simulink model "dvbs1_batch"  (R2024b)
settings: Solver=VariableStepDiscrete  StartTime=0.0  StopTime=inf  RelTol=1e-3  EnableMultiTasking=on
values from neighbouring files (symbols this model uses):
  EbNo = 3.3    [errPattern.m]    (also in symuluj_przeplot.m = 0:0.1:2.9)
  M = 4    [errPattern.m]    (also in wsp_szczytu.m)
undefined symbols (not defined in the file or in its folder): EbNodB, rsgenpoly
libraries: simulink x4, commsink2 x3, commdigbbndpm3 x3, commblkcod2 x2, commcnvcod2 x2, commcnvintrlv2 x2, commchan3 x1, commrandsrc2 x1
settings Model: Creator=Administrator  LastModifiedBy=mateu
settings SolverCC: AlgebraicLoopSolver=TrustRegion
settings DataIOCC: LimitDataPoints=on  SaveFormat=Array  SignalLoggingSaveFormat=ModelDataLogs  ReturnWorkspaceOutputs=off
settings OptimizationCC: ExpressionDepthLimit=2147483647  InitFltsAndDblsToZero=on  LifeSpan=inf
settings DebuggingCC: UnderspecifiedInitializationDetection=Classic  MergeDetectMultiDrivingBlocksExec=none  SolverPrmCheckMsg=warning  FcnCallInpInsideContextMsg=warning  UnconnectedInputMsg=warning  UnconnectedOutputMsg=warning  UnconnectedLineMsg=warning  StateNameClashWarn=warning  SFUnexpectedBacktrackingDiag=warning  SFNoUnconditionalDefaultTransitionDiag=warning  ArithmeticOperatorsInVariantConditions=warning
settings HardwareCC: ProdBitPerPointer=32  ProdBitPerSizeT=32  ProdBitPerPtrDiffT=32  ProdLargestAtomicFloat=None  ProdIntDivRoundTo=Undefined  ProdEndianess=Unspecified  ProdWordSize=32  ProdHWDeviceType=32-bit Generic
settings ModelReferenceCC: EnableRefExpFcnMdlSchedulingChecks=on  PropagateSignalLabelsOutOfModel=off
settings SFSimCC: SimUseLocalCustomCode=off  CustomCodeUndefinedFunction=UseInterfaceOnly
settings RTWCC: RTWUseLocalCustomCode=off  GPUComputeCapability=3.5
settings CodeAppCC: StateflowObjectComments=on
settings GRTTargetCC: TargetLangStandard=C89/C90 (ANSI)  CombineOutputUpdateFcns=off  GRTInterface=on
settings ConfigComp: CovMetricSettings=dw  CovSaveCumulativeToWorkspaceVar=on  CovSaveSingleToWorkspaceVar=on  CovExternalEMLEnable=off  CovSFcnEnable=off

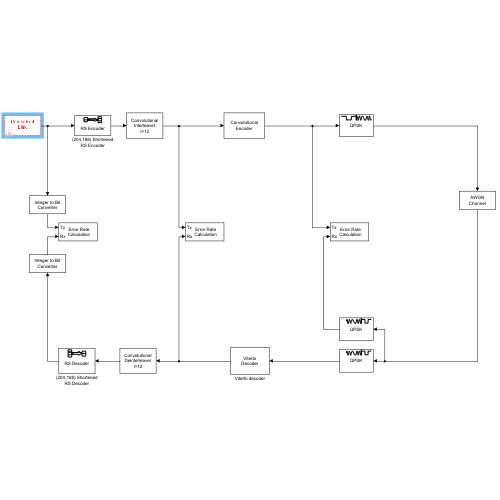
[thumbnail: Simulink's stored preview of the top-level diagram]
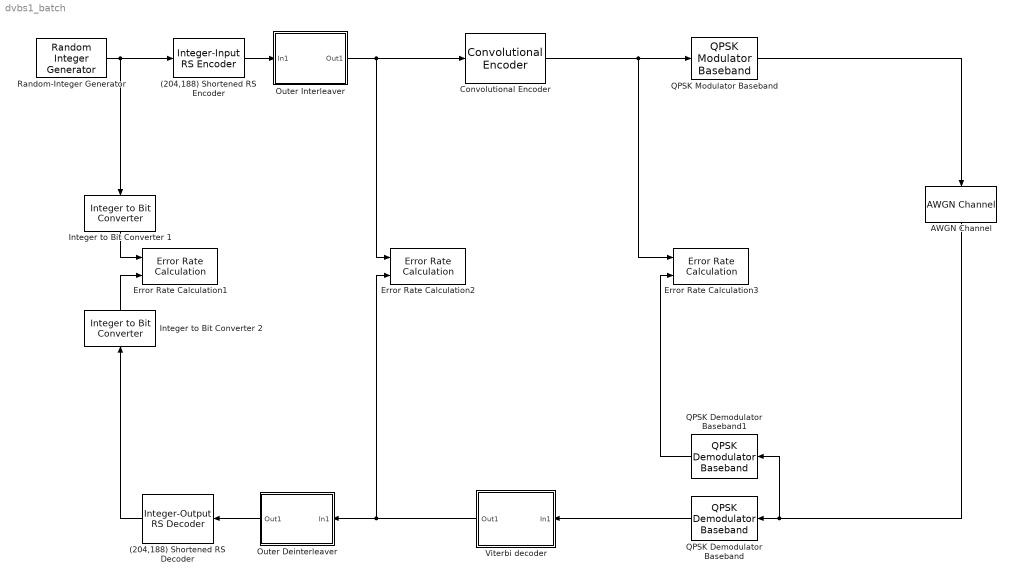
== system dvbs1_batch ==
  (204,188) Shortened RS Decoder : commblkcod2/Integer-Output RS Decoder  n=204  k=188  specShortening=off  shortenedK=3  specGenPoly=off  genPoly=rsgenpoly(7,3)  specPrimPoly=off  prPoly=[1 0 1 1]  specPuncture=off  punctVec=[ones(2,1); zeros(2,1)]  specErasurePort=off  showNumErr=off
  (204,188) Shortened RS Encoder : commblkcod2/Integer-Input RS Encoder  n=204  k=188  specShortening=off  shortenedK=3  specGenPoly=off  genPoly=rsgenpoly(7,3)  specPrimPoly=off  prPoly=[1 0 1 1]  specPuncture=off  punctVec=[ones(2,1); zeros(2,1)]
  AWGN Channel : commchan3/AWGN Channel  LegacyMode=on  NoiseMethod="Signal to noise ratio  (SNR)"  noiseMode="Signal to noise ratio  (SNR)"  EbNo=EbNo  EsNo=EbNodB+10*log10(log2(M))  SNR=EbNo + 1.20574  BitsPerSymbol=2  SignalPower=1  SamplesPerSymbol=1  SymbolPeriod=1.334  VarianceSource=Parameter  Variance=10^(-0.1*15)/(2048*2)  RandomStream=Global stream  Seed=54321  SimulateUsing=Code generation
  Convolutional Encoder : commcnvcod2/Convolutional Encoder  trellis=poly2trellis(7, [171 133])  opMode=Continuous  DelayedResetAction=off  hasIniStPort=off  hasFinStPort=off  usePuncVector=on  punctureVector=[1; 1; 0; 1]  reset=Unused parameter value
  Error Rate Calculation1 : commsink2/Error Rate Calculation  N=1504  st_delay=0  cp_mode=Entire frame  subframe=[]  PMode=Workspace  WsName=BerRs  RsMode2=off  stop=on  numErr=100  maxBits=1e7
  Error Rate Calculation2 : commsink2/Error Rate Calculation  N=1632  st_delay=0  cp_mode=Entire frame  subframe=[]  PMode=Workspace  WsName=BerFec  RsMode2=off  stop=off  numErr=100  maxBits=1e8
  Error Rate Calculation3 : commsink2/Error Rate Calculation  N=0  st_delay=0  cp_mode=Entire frame  subframe=[]  PMode=Workspace  WsName=BerRaw  RsMode2=off  stop=off  numErr=100  maxBits=1e8
  Integer to Bit Converter 1 : simulink/Logic and Bit Operations/Integer to Bit Converter  nbits=8  signedInputValues=Unsigned  bitOrder=MSB first  outDtype=boolean
  Integer to Bit Converter 2 : simulink/Logic and Bit Operations/Integer to Bit Converter  nbits=8  signedInputValues=Unsigned  bitOrder=MSB first  outDtype=boolean
  Outer Deinterleaver : Subsystem  mask(Convolutional Deinterleaver){}
      mask Display: disp('Convolutional\nDeinterleaver\nI=12')
  Outer Interleaver : Subsystem  mask(Convolutional Interleaver){}
      mask Display: disp('Convolutional\nInterleaver\nI=12')
  QPSK Demodulator Baseband : commdigbbndpm3/QPSK Demodulator Baseband  OutType=Bit  DecType=Approximate log-likelihood ratio  VarSource=Dialog  Variance=(1.0/(2*0.66))*10^(-EbNo/10)  Dec=Gray  Ph=pi/4  outDtype1=boolean  outDtype2=Inherit via internal rule  derotateFactorWordLen=16  derotateFactorDataTypeStr=Inherit: Same word length as input  derotateFactorLastDataTypeStr=Inherit: Same word length as input
  QPSK Demodulator Baseband1 : commdigbbndpm3/QPSK Demodulator Baseband  OutType=Bit  DecType=Hard decision  VarSource=Dialog  Variance=(1.0/(2*0.66))*10^(-EbNo/10)  Dec=Gray  Ph=pi/4  outDtype1=boolean  outDtype2=Inherit via internal rule  derotateFactorWordLen=16  derotateFactorDataTypeStr=Inherit: Same word length as input  derotateFactorLastDataTypeStr=Inherit: Same word length as input
  QPSK Modulator Baseband : commdigbbndpm3/QPSK Modulator Baseband  InType=Bit  Enc=Gray  Ph=pi/4  outDtype=double  outWordLen=16  outUDDataType=sfix(16)  outFracLenMode=Best precision  outFracLen=15  outDataTypeStr=double  outLastDataTypeStr=double
  Random-Integer Generator : commrandsrc2/Random Integer Generator  mul=256  seed=1234573  Ts=8*(204/188)  frameBased=on  sampPerFrame=188  orient=off  outDataType=uint8
  Viterbi decoder : Subsystem
      mask Display: disp('Viterbi\nDecoder')
  wires:
  (204,188) Shortened RS Encoder/1 -> Outer Interleaver/1(In1)
  Outer Interleaver/1(Out1) -> Convolutional Encoder/1, Error Rate Calculation2/1
  QPSK Modulator Baseband/1 -> AWGN Channel/1
  QPSK Demodulator Baseband/1 -> Viterbi decoder/1(In1)
  Outer Deinterleaver/1(Out1) -> (204,188) Shortened RS Decoder/1
  (204,188) Shortened RS Decoder/1 -> Integer to Bit Converter 2/1
  Convolutional Encoder/1 -> QPSK Modulator Baseband/1, Error Rate Calculation3/1
  Random-Integer Generator/1 -> (204,188) Shortened RS Encoder/1, Integer to Bit Converter 1/1
  Viterbi decoder/1(Out1) -> Outer Deinterleaver/1(In1), Error Rate Calculation2/2
  Integer to Bit Converter 1/1 -> Error Rate Calculation1/1
  Integer to Bit Converter 2/1 -> Error Rate Calculation1/2
  AWGN Channel/1 -> QPSK Demodulator Baseband1/1, QPSK Demodulator Baseband/1
  QPSK Demodulator Baseband1/1 -> Error Rate Calculation3/2

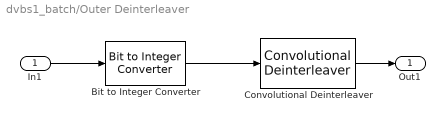
== system dvbs1_batch/Outer Deinterleaver ==
  In1 : Inport
  Bit to Integer Converter : simulink/Logic and Bit Operations/Bit to Integer Converter  nbits=8  bitOrder=MSB first  signedOutputValues=Unsigned  outDtype=uint8  outDtypeSigned=Inherit via internal rule
  Convolutional Deinterleaver : commcnvintrlv2/Convolutional Deinterleaver  N=1  B=204  ic=0
  Out1 : Outport
  wires:
  In1/1 -> Bit to Integer Converter/1
  Convolutional Deinterleaver/1 -> Out1/1
  Bit to Integer Converter/1 -> Convolutional Deinterleaver/1

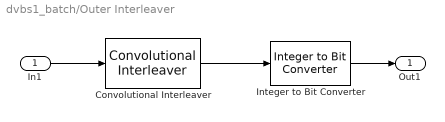
== system dvbs1_batch/Outer Interleaver ==
  In1 : Inport
  Convolutional Interleaver : commcnvintrlv2/Convolutional Interleaver  N=1  B=204  ic=0
  Integer to Bit Converter : simulink/Logic and Bit Operations/Integer to Bit Converter  nbits=8  signedInputValues=Unsigned  bitOrder=MSB first  outDtype=boolean
  Out1 : Outport
  wires:
  Integer to Bit Converter/1 -> Out1/1
  Convolutional Interleaver/1 -> Integer to Bit Converter/1
  In1/1 -> Convolutional Interleaver/1

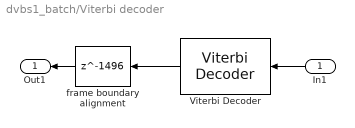
== system dvbs1_batch/Viterbi decoder ==
  In1 : Inport
  " frame boundary alignment" : Delay  DelayLength=1496  InitialCondition=0  InputProcessing=Columns as channels (frame based)
  Viterbi Decoder : commcnvcod2/Viterbi Decoder  trellis=poly2trellis(7, [171 133])  isPunctured=on  punctureVector=[1; 1; 0; 1]  erasures=off  dectype=Unquantized  nsdecb=4  runSigValErrCheck=off  tbdepth=136  opmode=Continuous  reset=off  delayedResetAction=off  smWordLength=16  outDataType=boolean
  Out1 : Outport
  wires:
  Viterbi Decoder/1 -> " frame boundary alignment"/1
  In1/1 -> Viterbi Decoder/1
  " frame boundary alignment"/1 -> Out1/1
